simulink model "EXAMPLE_1st_order_tf"  (R2022a)
settings: Solver=ode8  StartTime=0.0  StopTime=20  FixedStep=1/1000  RelTol=1e-3
undefined symbols (not defined in the file or in its folder): scale, sigbuilder_block
libraries: slpidlib x3
settings Model: Creator=martin  LastModifiedBy=martin

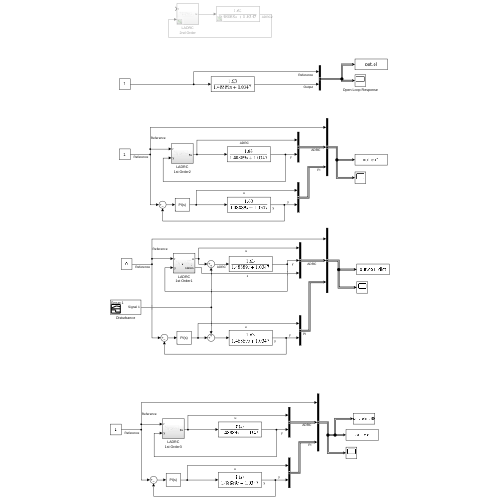
[thumbnail: Simulink's stored preview of the top-level diagram]
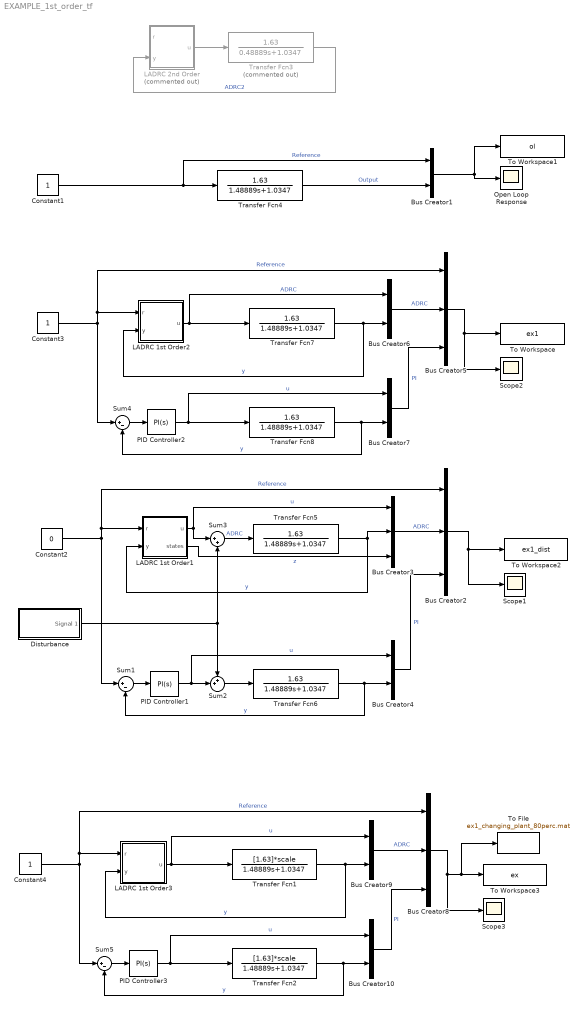
== system EXAMPLE_1st_order_tf ==
  Bus Creator{1,4,6..7,9..10} (6 alike) : BusCreator  Inputs=2
  Bus Creator{2..3,5,8} (4 alike) : BusCreator  Inputs=3
  Constant1 : Constant  VectorParams1D=off
  Constant2 : Constant  Value=0  VectorParams1D=off
  Constant3 : Constant  VectorParams1D=off
  Constant4 : Constant  VectorParams1D=off
  Disturbance : Subsystem  Tag=STV Subsys  LoadFcn=sigbuilder_block('load');  StartFcn=sigbuilder_block('start');  StopFcn=sigbuilder_block('stop');  ClipboardFcn=sigbuilder_block('clipboard');  mask(Sigbuilder block){tuvar=[0:10]}
      mask help: Simulink:masks:SigbuilderBlock_MD
      mask init:
      | if ~strcmp(get_param(bdroot(gcbh),'SimulationStatus'),'stopped') tuvar = sigbuilder_block('maskInit'); end
      settings: CopyFcn=sigbuilder_block('copy');  DeleteFcn=sigbuilder_block('delete');  ModelCloseFcn=sigbuilder_block('modelClose');  PreSaveFcn=sigbuilder_block('preSave');  PauseFcn=sigbuilder_block('pause');  ContinueFcn=sigbuilder_block('continue');  NameChangeFcn=sigbuilder_block('namechange');  OpenFcn=sigbuilder_block('open',[323.644 160.396 557.465 395.644 ]);  CloseFcn=sigbuilder_block('close');
      mask Display: plot(0, 0, 100, 100,[2, 2, 32, 32, 2], [68, 8, 8, 68, 68],[32, 2], [38, 38], [32, 19, 2],[53, 60, 44], [32, 17, 17, 2],[16, 16, 31, 31]);txt = getActiveGroup(gcbh);text(2, 100, txt,'verticalAlignment', 'top');
  LADRC 1st Order1 : Subsystem  VariantControl=Choice
  LADRC 1st Order2 : Subsystem  VariantControl=Choice
  LADRC 1st Order3 : Subsystem  VariantControl=Choice
  LADRC 2nd Order : Subsystem  Commented=on  VariantControl=Choice
  Open Loop Response : Scope
  PID Controller1 : slpidlib/PID Controller  Controller=PI  Form=Parallel  TimeDomain=Continuous-time  UseExternalTs=off  SampleTime=-1  IntegratorMethod=Forward Euler  FilterMethod=Forward Euler  ControllerParametersSource=internal  P=2.74028834355828  I=1.90435582822086  UseKiTs=off  D=0.0374613983911996  N=6.88177099897913  UseFilter=on  TunerSelectOption=Transfer Function Based (PID Tuner App)  InitialConditionSource=internal  InitialConditionForIntegrator=0  InitialConditionForFilter=0  DifferentiatorICPrevScaledInput=0  ExternalReset=none  TrackingMode=off  Kt=1  LimitOutput=off  SatLimitsSource=internal  UpperSaturationLimit=inf  LowerSaturationLimit=-inf  LinearizeAsGain=on  AntiWindupMode=none  Kb=1  POutMin=[]  POutMax=[]  IOutMin=[]  IOutMax=[]  DOutMin=[]  DOutMax=[]  NOutMin=[]  NOutMax=[]  SumOutMin=[]  SumOutMax=[]  SaturationOutMin=[]  SaturationOutMax=[]  PParamMin=[]  PParamMax=[]  IParamMin=[]  IParamMax=[]  DParamMin=[]  DParamMax=[]  NParamMin=[]  NParamMax=[]  KbParamMin=[]  KbParamMax=[]  KtParamMin=[]  KtParamMax=[]  KbOutMin=[]  KbOutMax=[]  KtOutMin=[]  KtOutMax=[]  IntegratorOutMin=[]  IntegratorOutMax=[]  FilterOutMin=[]  FilterOutMax=[]  SumI1OutMin=[]  SumI1OutMax=[]  SumI2OutMin=[]  SumI2OutMax=[]  SumI3OutMin=[]  SumI3OutMax=[]  SumI4OutMin=[]  SumI4OutMax=[]  SumDOutMin=[]  SumDOutMax=[]  DifferentiatorOutMin=[]  DifferentiatorOutMax=[]  FilterDiffOutCoefMin=[]  FilterDiffOutCoefMax=[]  ReciprocalOutMin=[]  ReciprocalOutMax=[]  SumDenOutMin=[]  SumDenOutMax=[]  SumNumOutMin=[]  SumNumOutMax=[]  DivideOutMin=[]  DivideOutMax=[]  UdiffTsProdOutMin=[]  UdiffTsProdOutMax=[]  NTsProdOutMin=[]  NTsProdOutMax=[]  UintegralTsProdOutMin=[]  UintegralTsProdOutMax=[]  UngainTsProdOutMin=[]  UngainTsProdOutMax=[]  IntegratorContinuousStateAttributes=''  IntegratorStateMustResolveToSignalObject=off  IntegratorRTWStateStorageClass=Auto  FilterContinuousStateAttributes=''  FilterStateMustResolveToSignalObject=off  FilterRTWStateStorageClass=Auto  ParallelPVariant=InternalParameters  IdealPVariant=Disabled  IVariant=InternalParameters  DVariant=Disabled  IntegratorVariant=Continuous  SatVariant=Disabled  AWVariant=Passthrough  PCopyVariant=Disabled  TRVariant=Disabled  FdbkBlocksVariant=Forward  IdealPFdbkVariant=Disabled  SatFdbkVariant=Disabled  DerivativeFilterVariant=Disabled  NVariant=Disabled  NCopyVariant=Disabled_SignalSpec  FilterICVariant=Disabled  IntegratorICVariant=InternalICs  ExternalResetVariant=Disabled  TRSumVariant=Passthrough  SumFdbkVariant=Disabled  SumVariant=Sum_PI  TsampFilterVariant=InternalTs  TsampNgainVariant=Passthrough  TsampIntegralVariant=Passthrough  ExternalSaturationOutDataTypeStr=Inherit: Same as second input  aMode=0
  PID Controller2 : slpidlib/PID Controller  Controller=PI  Form=Parallel  TimeDomain=Continuous-time  UseExternalTs=off  SampleTime=-1  IntegratorMethod=Forward Euler  FilterMethod=Forward Euler  ControllerParametersSource=internal  P=2.74028834355828  I=1.90435582822086  UseKiTs=off  D=0.0374613983911996  N=6.88177099897913  UseFilter=on  TunerSelectOption=Transfer Function Based (PID Tuner App)  InitialConditionSource=internal  InitialConditionForIntegrator=0  InitialConditionForFilter=0  DifferentiatorICPrevScaledInput=0  ExternalReset=none  TrackingMode=off  Kt=1  LimitOutput=off  SatLimitsSource=internal  UpperSaturationLimit=inf  LowerSaturationLimit=-inf  LinearizeAsGain=on  AntiWindupMode=none  Kb=1  POutMin=[]  POutMax=[]  IOutMin=[]  IOutMax=[]  DOutMin=[]  DOutMax=[]  NOutMin=[]  NOutMax=[]  SumOutMin=[]  SumOutMax=[]  SaturationOutMin=[]  SaturationOutMax=[]  PParamMin=[]  PParamMax=[]  IParamMin=[]  IParamMax=[]  DParamMin=[]  DParamMax=[]  NParamMin=[]  NParamMax=[]  KbParamMin=[]  KbParamMax=[]  KtParamMin=[]  KtParamMax=[]  KbOutMin=[]  KbOutMax=[]  KtOutMin=[]  KtOutMax=[]  IntegratorOutMin=[]  IntegratorOutMax=[]  FilterOutMin=[]  FilterOutMax=[]  SumI1OutMin=[]  SumI1OutMax=[]  SumI2OutMin=[]  SumI2OutMax=[]  SumI3OutMin=[]  SumI3OutMax=[]  SumI4OutMin=[]  SumI4OutMax=[]  SumDOutMin=[]  SumDOutMax=[]  DifferentiatorOutMin=[]  DifferentiatorOutMax=[]  FilterDiffOutCoefMin=[]  FilterDiffOutCoefMax=[]  ReciprocalOutMin=[]  ReciprocalOutMax=[]  SumDenOutMin=[]  SumDenOutMax=[]  SumNumOutMin=[]  SumNumOutMax=[]  DivideOutMin=[]  DivideOutMax=[]  UdiffTsProdOutMin=[]  UdiffTsProdOutMax=[]  NTsProdOutMin=[]  NTsProdOutMax=[]  UintegralTsProdOutMin=[]  UintegralTsProdOutMax=[]  UngainTsProdOutMin=[]  UngainTsProdOutMax=[]  IntegratorContinuousStateAttributes=''  IntegratorStateMustResolveToSignalObject=off  IntegratorRTWStateStorageClass=Auto  FilterContinuousStateAttributes=''  FilterStateMustResolveToSignalObject=off  FilterRTWStateStorageClass=Auto  ParallelPVariant=InternalParameters  IdealPVariant=Disabled  IVariant=InternalParameters  DVariant=Disabled  IntegratorVariant=Continuous  SatVariant=Disabled  AWVariant=Passthrough  PCopyVariant=Disabled  TRVariant=Disabled  FdbkBlocksVariant=Forward  IdealPFdbkVariant=Disabled  SatFdbkVariant=Disabled  DerivativeFilterVariant=Disabled  NVariant=Disabled  NCopyVariant=Disabled_SignalSpec  FilterICVariant=Disabled  IntegratorICVariant=InternalICs  ExternalResetVariant=Disabled  TRSumVariant=Passthrough  SumFdbkVariant=Disabled  SumVariant=Sum_PI  TsampFilterVariant=InternalTs  TsampNgainVariant=Passthrough  TsampIntegralVariant=Passthrough  ExternalSaturationOutDataTypeStr=Inherit: Same as second input  aMode=0
  PID Controller3 : slpidlib/PID Controller  Controller=PI  Form=Parallel  TimeDomain=Continuous-time  UseExternalTs=off  SampleTime=-1  IntegratorMethod=Forward Euler  FilterMethod=Forward Euler  ControllerParametersSource=internal  P=2.74028834355828  I=1.90435582822086  UseKiTs=off  D=0.0374613983911996  N=6.88177099897913  UseFilter=on  TunerSelectOption=Transfer Function Based (PID Tuner App)  InitialConditionSource=internal  InitialConditionForIntegrator=0  InitialConditionForFilter=0  DifferentiatorICPrevScaledInput=0  ExternalReset=none  TrackingMode=off  Kt=1  LimitOutput=off  SatLimitsSource=internal  UpperSaturationLimit=inf  LowerSaturationLimit=-inf  LinearizeAsGain=on  AntiWindupMode=none  Kb=1  POutMin=[]  POutMax=[]  IOutMin=[]  IOutMax=[]  DOutMin=[]  DOutMax=[]  NOutMin=[]  NOutMax=[]  SumOutMin=[]  SumOutMax=[]  SaturationOutMin=[]  SaturationOutMax=[]  PParamMin=[]  PParamMax=[]  IParamMin=[]  IParamMax=[]  DParamMin=[]  DParamMax=[]  NParamMin=[]  NParamMax=[]  KbParamMin=[]  KbParamMax=[]  KtParamMin=[]  KtParamMax=[]  KbOutMin=[]  KbOutMax=[]  KtOutMin=[]  KtOutMax=[]  IntegratorOutMin=[]  IntegratorOutMax=[]  FilterOutMin=[]  FilterOutMax=[]  SumI1OutMin=[]  SumI1OutMax=[]  SumI2OutMin=[]  SumI2OutMax=[]  SumI3OutMin=[]  SumI3OutMax=[]  SumI4OutMin=[]  SumI4OutMax=[]  SumDOutMin=[]  SumDOutMax=[]  DifferentiatorOutMin=[]  DifferentiatorOutMax=[]  FilterDiffOutCoefMin=[]  FilterDiffOutCoefMax=[]  ReciprocalOutMin=[]  ReciprocalOutMax=[]  SumDenOutMin=[]  SumDenOutMax=[]  SumNumOutMin=[]  SumNumOutMax=[]  DivideOutMin=[]  DivideOutMax=[]  UdiffTsProdOutMin=[]  UdiffTsProdOutMax=[]  NTsProdOutMin=[]  NTsProdOutMax=[]  UintegralTsProdOutMin=[]  UintegralTsProdOutMax=[]  UngainTsProdOutMin=[]  UngainTsProdOutMax=[]  IntegratorContinuousStateAttributes=''  IntegratorStateMustResolveToSignalObject=off  IntegratorRTWStateStorageClass=Auto  FilterContinuousStateAttributes=''  FilterStateMustResolveToSignalObject=off  FilterRTWStateStorageClass=Auto  ParallelPVariant=InternalParameters  IdealPVariant=Disabled  IVariant=InternalParameters  DVariant=Disabled  IntegratorVariant=Continuous  SatVariant=Disabled  AWVariant=Passthrough  PCopyVariant=Disabled  TRVariant=Disabled  FdbkBlocksVariant=Forward  IdealPFdbkVariant=Disabled  SatFdbkVariant=Disabled  DerivativeFilterVariant=Disabled  NVariant=Disabled  NCopyVariant=Disabled_SignalSpec  FilterICVariant=Disabled  IntegratorICVariant=InternalICs  ExternalResetVariant=Disabled  TRSumVariant=Passthrough  SumFdbkVariant=Disabled  SumVariant=Sum_PI  TsampFilterVariant=InternalTs  TsampNgainVariant=Passthrough  TsampIntegralVariant=Passthrough  ExternalSaturationOutDataTypeStr=Inherit: Same as second input  aMode=0
  Scope1 : Scope
  Scope2 : Scope
  Scope3 : Scope
  Sum1 : Sum  Inputs=|+-
  Sum2 : Sum  Inputs=++|
  Sum3 : Sum  Inputs=|++
  Sum4 : Sum  Inputs=|+-
  Sum5 : Sum  Inputs=|+-
  To File : ToFile  Filename=ex1_changing_plant_80perc.mat  SaveFormat=Timeseries
  To Workspace : ToWorkspace  VariableName=ex1  SaveFormat=Timeseries  SampleTime=-1
  To Workspace1 : ToWorkspace  VariableName=ol  SaveFormat=Timeseries  SampleTime=-1
  To Workspace2 : ToWorkspace  VariableName=ex1_dist  SaveFormat=Timeseries  SampleTime=-1
  To Workspace3 : ToWorkspace  VariableName=ex  SaveFormat=Timeseries  SampleTime=-1
  Transfer Fcn1 : TransferFcn  Numerator=[1.63]*scale  Denominator=[1.48889 1.0347]
  Transfer Fcn2 : TransferFcn  Numerator=[1.63]*scale  Denominator=[1.48889 1.0347]
  Transfer Fcn3 : TransferFcn  Commented=on  Numerator=[1.63]  Denominator=[0.48889 1.0347]
  Transfer Fcn{4..8} (5 alike) : TransferFcn  Numerator=[1.63]  Denominator=[1.48889 1.0347]
  wires:
  LADRC 2nd Order/1(u) -> Transfer Fcn3/1
  Transfer Fcn3/1 -> LADRC 2nd Order/2(y)  "ADRC2"
  Transfer Fcn4/1 -> Bus Creator1/2  "Output"
  Bus Creator1/1 -> To Workspace1/1, Open Loop Response/1
  Constant1/1 -> Bus Creator1/1, Transfer Fcn4/1  "Reference"
  Sum1/1 -> PID Controller1/1
  Constant2/1 -> Bus Creator2/1, LADRC 1st Order1/1(r), Sum1/1  "Reference"
  Bus Creator2/1 -> Scope1/1, To Workspace2/1
  LADRC 1st Order1/1(u) -> Sum3/1, Bus Creator3/1  "u"
  Transfer Fcn6/1 -> Bus Creator4/2, Sum1/2  "y"
  Disturbance/1(Signal 1) -> Sum3/2, Sum2/1
  Transfer Fcn5/1 -> Bus Creator3/2, LADRC 1st Order1/2(y)  "y"
  Sum3/1 -> Transfer Fcn5/1  "ADRC"
  Sum2/1 -> Transfer Fcn6/1
  PID Controller1/1 -> Bus Creator4/1, Sum2/2  "u"
  Bus Creator3/1 -> Bus Creator2/2  "ADRC"
  Bus Creator4/1 -> Bus Creator2/3  "PI"
  Transfer Fcn7/1 -> Bus Creator6/2, LADRC 1st Order2/2(y)  "y"
  Bus Creator7/1 -> Bus Creator5/3  "PI"
  LADRC 1st Order2/1(u) -> Transfer Fcn7/1, Bus Creator6/1  "ADRC"
  PID Controller2/1 -> Transfer Fcn8/1, Bus Creator7/1  "u"
  Transfer Fcn8/1 -> Bus Creator7/2, Sum4/2  "y"
  Bus Creator6/1 -> Bus Creator5/2  "ADRC"
  Sum4/1 -> PID Controller2/1
  Bus Creator5/1 -> Scope2/1, To Workspace/1
  Constant3/1 -> Bus Creator5/1, LADRC 1st Order2/1(r), Sum4/1  "Reference"
  LADRC 1st Order1/2(states) -> Bus Creator3/3  "z"
  LADRC 1st Order3/1(u) -> Transfer Fcn1/1, Bus Creator9/1  "u"
  Bus Creator9/1 -> Bus Creator8/2  "ADRC"
  PID Controller3/1 -> Transfer Fcn2/1, Bus Creator10/1  "u"
  Bus Creator10/1 -> Bus Creator8/3  "PI"
  Transfer Fcn1/1 -> Bus Creator9/2, LADRC 1st Order3/2(y)  "y"
  Bus Creator8/1 -> Scope3/1, To File/1, To Workspace3/1
  Transfer Fcn2/1 -> Bus Creator10/2, Sum5/2  "y"
  Sum5/1 -> PID Controller3/1
  Constant4/1 -> Bus Creator8/1, LADRC 1st Order3/1(r), Sum5/1  "Reference"

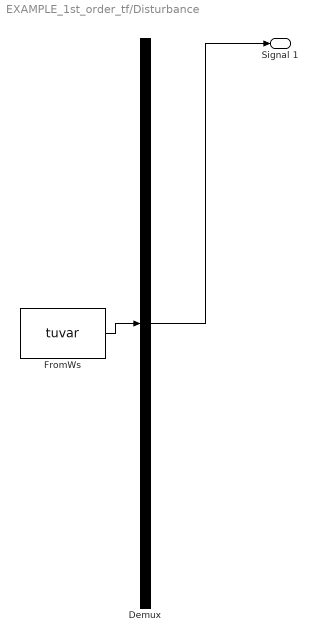
== system EXAMPLE_1st_order_tf/Disturbance ==
  Demux : Demux  Tag=STV Demux  Outputs=1
      settings: DisplayOption=none
  FromWs : FromWorkspace  Tag=STV FromWs  VariableName=tuvar
      SigBuilderData=|
      | common.afterFinalStr = 'Extrapolate'
      | common.sampleTime = 0
      | dataSet.timeRange = [0 100]
      | dataSet.name = 'Group 1'
      | sbobj.Groups.Name = 'Group 1'
      | sbobj.Groups.Signals.Name = 'Signal 1'
      | sbobj.Groups.Signals.XData = [0 5 5 10 10 100]
      | sbobj.Groups.Signals.YData = [0 0 1.5 1.5 0 0]
      | sbobj.Groups.TimeRange = [0 100]
  Signal 1 : Outport  Tag=STV Outport
  wires:
  Demux/1 -> Signal 1/1
  FromWs/1 -> Demux/1

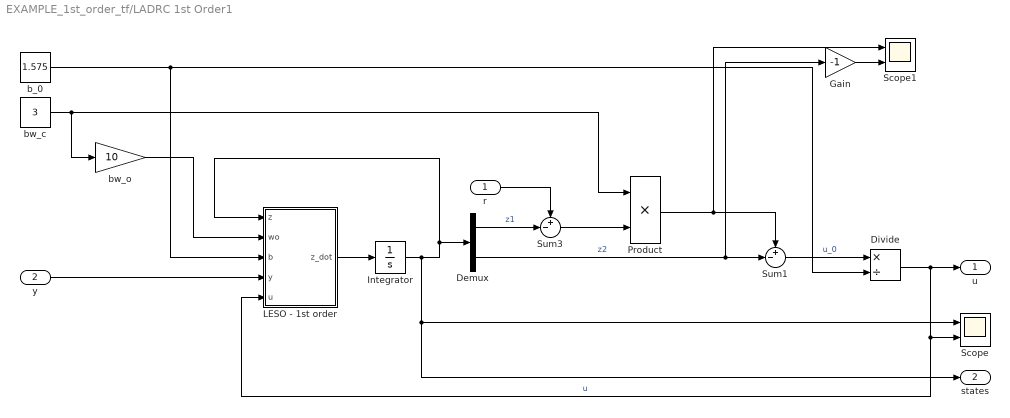
== system EXAMPLE_1st_order_tf/LADRC 1st Order1 ==
  r : Inport
  y : Inport  Port=2
  Demux : Demux  Outputs=2
  Divide : Product  Inputs=*/
  Gain : Gain  Gain=-1
  Integrator : Integrator  InitialCondition=[0 0]'
  LESO - 1st order : MATLAB Function  TreatAsAtomicUnit=on
  Product : Product
  Scope : Scope  NumInputPorts=2
  Scope1 : Scope  NumInputPorts=2
  Sum1 : Sum  Inputs=+-|
  Sum3 : Sum  Inputs=+-|
  b_0 : Constant  Value=1.575
  bw_c : Constant  Value=3
  bw_o : Gain  Gain=10
  u : Outport
  states : Outport  Port=2
  wires:
  LESO - 1st order/1(z_dot) -> Integrator/1
  Integrator/1 -> states/1, Scope/1, LESO - 1st order/1(z), Demux/1
  Demux/1 -> Sum3/2  "z1"
  Product/1 -> Scope1/1, Sum1/1
  Sum1/1 -> Divide/1  "u_0"
  Demux/2 -> Gain/1, Sum1/2  "z2"
  Divide/1 -> u/1, Scope/2, LESO - 1st order/5(u)  "u"
  r/1 -> Sum3/1
  Sum3/1 -> Product/2
  b_0/1 -> LESO - 1st order/3(b), Divide/2
  bw_c/1 -> bw_o/1, Product/1
  bw_o/1 -> LESO - 1st order/2(wo)
  y/1 -> LESO - 1st order/4(y)
  Gain/1 -> Scope1/2

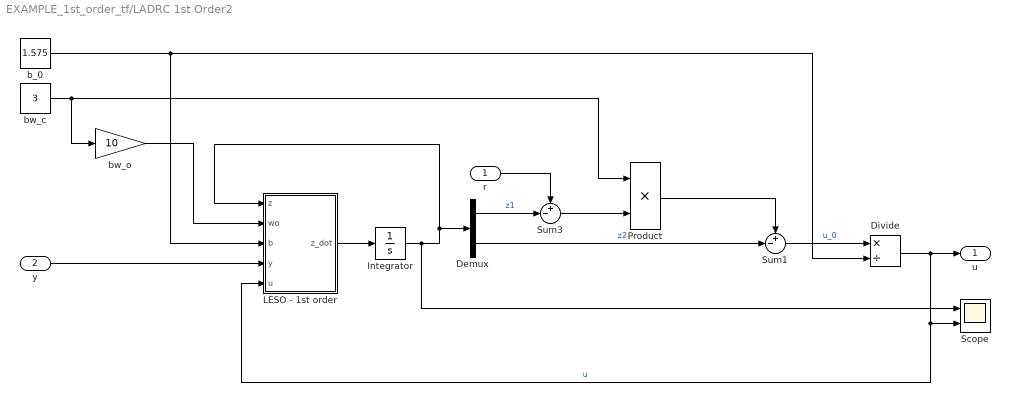
== system EXAMPLE_1st_order_tf/LADRC 1st Order2 ==
  r : Inport
  y : Inport  Port=2
  Demux : Demux  Outputs=2
  Divide : Product  Inputs=*/
  Integrator : Integrator  InitialCondition=[0 0]'
  LESO - 1st order : MATLAB Function  TreatAsAtomicUnit=on
  Product : Product
  Scope : Scope  NumInputPorts=2
  Sum1 : Sum  Inputs=+-|
  Sum3 : Sum  Inputs=+-|
  b_0 : Constant  Value=1.575
  bw_c : Constant  Value=3
  bw_o : Gain  Gain=10
  u : Outport
  wires:
  LESO - 1st order/1(z_dot) -> Integrator/1
  Integrator/1 -> Scope/1, LESO - 1st order/1(z), Demux/1
  Demux/1 -> Sum3/2  "z1"
  Product/1 -> Sum1/1
  Sum1/1 -> Divide/1  "u_0"
  Demux/2 -> Sum1/2  "z2"
  Divide/1 -> u/1, Scope/2, LESO - 1st order/5(u)  "u"
  r/1 -> Sum3/1
  Sum3/1 -> Product/2
  b_0/1 -> LESO - 1st order/3(b), Divide/2
  bw_c/1 -> bw_o/1, Product/1
  bw_o/1 -> LESO - 1st order/2(wo)
  y/1 -> LESO - 1st order/4(y)

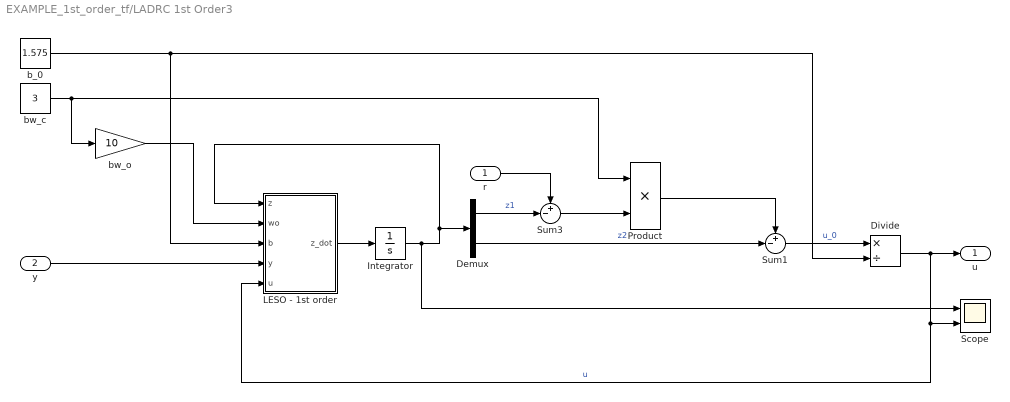
== system EXAMPLE_1st_order_tf/LADRC 1st Order3 ==
  r : Inport
  y : Inport  Port=2
  Demux : Demux  Outputs=2
  Divide : Product  Inputs=*/
  Integrator : Integrator  InitialCondition=[0 0]'
  LESO - 1st order : MATLAB Function  TreatAsAtomicUnit=on
  Product : Product
  Scope : Scope  NumInputPorts=2
  Sum1 : Sum  Inputs=+-|
  Sum3 : Sum  Inputs=+-|
  b_0 : Constant  Value=1.575
  bw_c : Constant  Value=3
  bw_o : Gain  Gain=10
  u : Outport
  wires:
  LESO - 1st order/1(z_dot) -> Integrator/1
  Integrator/1 -> Scope/1, LESO - 1st order/1(z), Demux/1
  Demux/1 -> Sum3/2  "z1"
  Product/1 -> Sum1/1
  Sum1/1 -> Divide/1  "u_0"
  Demux/2 -> Sum1/2  "z2"
  Divide/1 -> u/1, Scope/2, LESO - 1st order/5(u)  "u"
  r/1 -> Sum3/1
  Sum3/1 -> Product/2
  b_0/1 -> LESO - 1st order/3(b), Divide/2
  bw_c/1 -> bw_o/1, Product/1
  bw_o/1 -> LESO - 1st order/2(wo)
  y/1 -> LESO - 1st order/4(y)

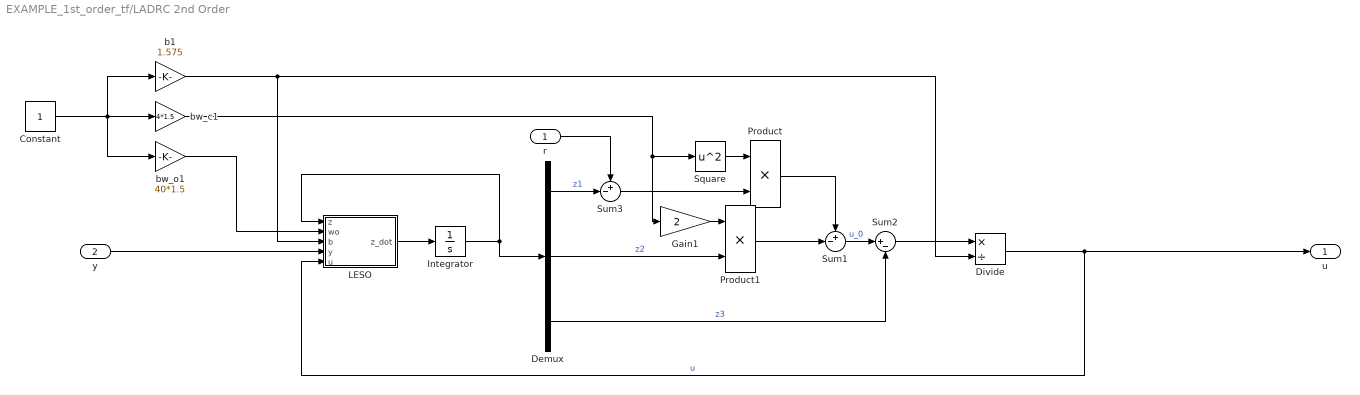
== system EXAMPLE_1st_order_tf/LADRC 2nd Order ==
  r : Inport
  y : Inport  Port=2
  Constant : Constant
  Demux : Demux  Outputs=3
  Divide : Product  Inputs=*/
  Gain1 : Gain  Gain=2
  Integrator : Integrator  InitialCondition=[0 0 0]'
  LESO : MATLAB Function  TreatAsAtomicUnit=on
  Product : Product
  Product1 : Product
  Square : Math  Operator=square
  Sum1 : Sum  Inputs=+-|
  Sum2 : Sum  Inputs=|+-
  Sum3 : Sum  Inputs=+-|
  b1 : Gain  Gain=1.575
  bw_c1 : Gain  Gain=4*1.5
  bw_o1 : Gain  Gain=40*1.5
  u : Outport
  wires:
  LESO/1(z_dot) -> Integrator/1
  Integrator/1 -> LESO/1(z), Demux/1
  Demux/1 -> Sum3/2  "z1"
  Product/1 -> Sum1/1
  Sum1/1 -> Sum2/1  "u_0"
  Demux/3 -> Sum2/2  "z3"
  Sum2/1 -> Divide/1
  Square/1 -> Product/1
  Gain1/1 -> Product1/1
  Demux/2 -> Product1/2  "z2"
  Product1/1 -> Sum1/2
  r/1 -> Sum3/1
  Sum3/1 -> Product/2
  b1/1 -> Divide/2, LESO/3(b)
  bw_c1/1 -> Gain1/1, Square/1
  bw_o1/1 -> LESO/2(wo)
  y/1 -> LESO/4(y)
  Constant/1 -> bw_o1/1, bw_c1/1, b1/1
  Divide/1 -> LESO/5(u), u/1  "u"

== matlab function EXAMPLE_1st_order_tf/LADRC 1st Order1/LESO - 1st order ==
  data: z input; wo input; b input; z_dot output; y input; u input
function z_dot = LESO(z, wo, b, y, u)
    A = [0 1; 0 0];
    B = [b 0]';
    L = [2*wo wo^2]';
        
    z_dot = A*z+ B*u + L*(y-z(1));

== matlab function EXAMPLE_1st_order_tf/LADRC 1st Order2/LESO - 1st order ==
  data: z input; wo input; b input; z_dot output; y input; u input
function z_dot = LESO(z, wo, b, y, u)
    A = [0 1; 0 0];
    B = [b 0]';
    L = [2*wo wo^2]';
        
    z_dot = A*z+ B*u + L*(y-z(1));

== matlab function EXAMPLE_1st_order_tf/LADRC 1st Order3/LESO - 1st order ==
  data: z input; wo input; b input; z_dot output; y input; u input
function z_dot = LESO(z, wo, b, y, u)
    A = [0 1; 0 0];
    B = [b 0]';
    L = [2*wo wo^2]';
        
    z_dot = A*z+ B*u + L*(y-z(1));

== matlab function EXAMPLE_1st_order_tf/LADRC 2nd Order/LESO ==
  data: z input; wo input; b input; z_dot output; y input; u input
function z_dot = LESO(z, wo, b, y, u)
    A = [0 1 0; 0 0 1; 0 0 0];
    B = [0 b 0]';
    C = [1 0 0];
    L = [3*wo 3*wo^2 wo^3]';
        
    z_dot = (A*z + B*u + L*(y-C*z));
